simulink model "System_1_5"  (R2017a)
settings: Solver=VariableStepAuto  StartTime=0.0  StopTime=1000  MaxStep=0.01  RelTol=1e-3
values from neighbouring files (symbols this model uses):
  k_k = double(vpasolve(eqn, kk))    [System1.m]
  r_t = b    (= 5)    [System1.m]
libraries: cstblocks x2
settings Model: Creator=dplascen  LastModifiedBy=dplascen
settings HardwareCC: ProdBitPerPointer=32  ProdBitPerSizeT=32  ProdBitPerPtrDiffT=32  ProdWordSize=32  ProdHWDeviceType=Intel->x86-32 (Windows32)

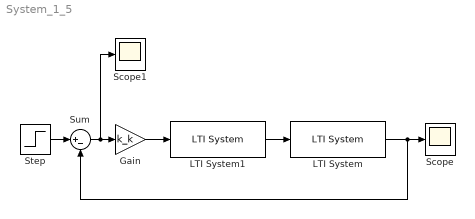
== system System_1_5 ==
  Gain : Gain  Gain=k_k
  LTI System : cstblocks/LTI System  sys=G  IC=[]
  LTI System1 : cstblocks/LTI System  sys=c_s  IC=[]
  Scope : Scope
  Scope1 : Scope
  Step : Step  Time=0  After=r_t  SampleTime=0
  Sum : Sum  Inputs=|+-
  wires:
  LTI System/1 -> Scope/1, Sum/2
  LTI System1/1 -> LTI System/1
  Step/1 -> Sum/1
  Sum/1 -> Scope1/1, Gain/1
  Gain/1 -> LTI System1/1
